simulink model "Mrac_MITS"  (R2015a)
settings: Solver=ode4  StartTime=to  StopTime=tf  FixedStep=dt  RelTol=1e-3
values from neighbouring files (symbols this model uses):
  G = 1/(s+1)    [MRAC_MIT.m]
  gamma1 = 0.5    [MRAC_MIT.m]
  gamma2 = 1    [MRAC_MIT.m]
  gamma3 = 2    [MRAC_MIT.m]
  k = 10* rand(1,length(t))    [MRAC_MIT.m]
libraries: cstblocks x6
settings Model: Creator=dj  LastModifiedBy=dj

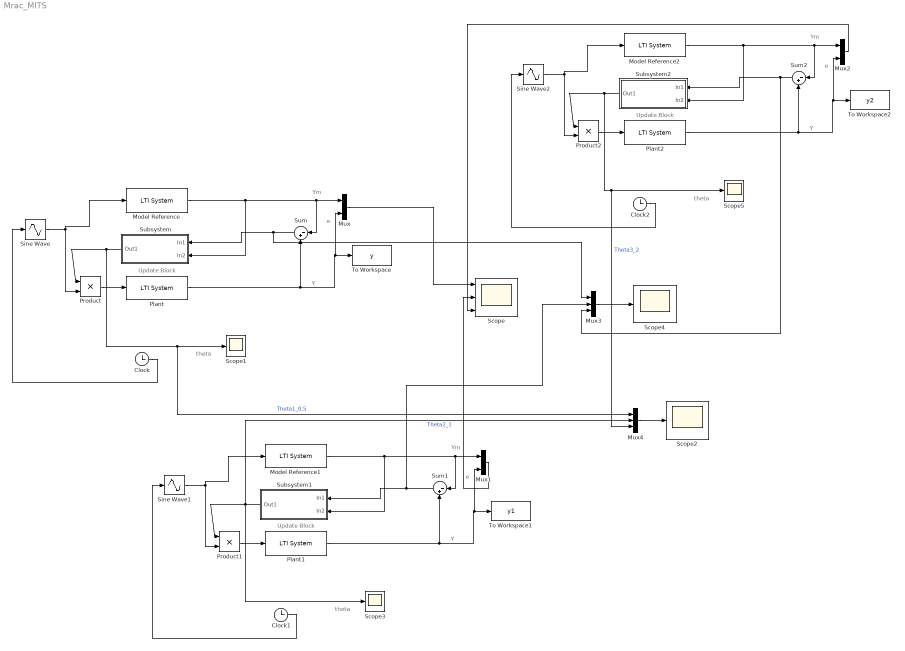
== system Mrac_MITS ==
  note: e
  note: Y
  note: Ym
  note: theta
  note: Update Block
  note: e
  note: Y
  note: Ym
  note: theta
  note: Update Block
  note: e
  note: Y
  note: Ym
  note: theta
  note: Update Block
  Clock : Clock
  Clock1 : Clock
  Clock2 : Clock
  Model Reference : cstblocks/LTI System  sys=Gm  IC=[]
  Model Reference1 : cstblocks/LTI System  sys=Gm  IC=[]
  Model Reference2 : cstblocks/LTI System  sys=Gm  IC=[]
  Mux : Mux  Inputs=2
  Mux1 : Mux  Inputs=2
  Mux2 : Mux  Inputs=2
  Mux3 : Mux  Inputs=3
  Mux4 : Mux  Inputs=3
  Plant : cstblocks/LTI System  sys=k*G  IC=[]
  Plant1 : cstblocks/LTI System  sys=k*G  IC=[]
  Plant2 : cstblocks/LTI System  sys=k*G  IC=[]
  Product : Product
  Product1 : Product
  Product2 : Product
  Scope : Scope  NumInputPorts=3
      settings: YMin=-5~-5~-5  YMax=5~5~5
  Scope{1..5} (5 alike) : Scope
      Scope2 settings: SaveName=ScopeData2
      Scope3 settings: SaveName=ScopeData3
      Scope4 settings: SaveName=ScopeData4
      Scope5 settings: SaveName=ScopeData5
  Sine Wave : Sin  TimeSource=Use external signal  SampleTime=0
  Sine Wave1 : Sin  TimeSource=Use external signal  SampleTime=0
  Sine Wave2 : Sin  TimeSource=Use external signal  SampleTime=0
  Subsystem : Subsystem
  Subsystem1 : Subsystem
  Subsystem2 : Subsystem
  Sum : Sum  Inputs=|-+
  Sum1 : Sum  Inputs=|-+
  Sum2 : Sum  Inputs=|-+
  To Workspace : ToWorkspace  VariableName=y  SaveFormat=Timeseries  SampleTime=-1
  To Workspace1 : ToWorkspace  VariableName=y1  SaveFormat=Timeseries  SampleTime=-1
  To Workspace2 : ToWorkspace  VariableName=y2  SaveFormat=Timeseries  SampleTime=-1
  wires:
  Model Reference/1 -> Subsystem/2(In2), Mux/1, Sum/1
  Product/1 -> Plant/1
  Subsystem/1(Out1) -> Mux4/1, Scope1/1, Product/1  "Theta1_0.5"
  Sum/1 -> Mux3/1, Subsystem/1(In1)
  Sine Wave/1 -> Model Reference/1, Product/2
  Plant/1 -> Mux/2, To Workspace/1, Sum/2
  Clock/1 -> Sine Wave/1
  Model Reference1/1 -> Subsystem1/2(In2), Mux1/1, Sum1/1
  Product1/1 -> Plant1/1
  Subsystem1/1(Out1) -> Mux4/2, Scope3/1, Product1/1  "Theta2_1"
  Sum1/1 -> Mux3/2, Subsystem1/1(In1)
  Sine Wave1/1 -> Model Reference1/1, Product1/2
  Plant1/1 -> Mux1/2, To Workspace1/1, Sum1/2
  Clock1/1 -> Sine Wave1/1
  Model Reference2/1 -> Sum2/1, Mux2/1, Subsystem2/2(In2)
  Product2/1 -> Plant2/1
  Subsystem2/1(Out1) -> Product2/1, Mux4/3, Scope5/1  "Theta3_2"
  Sum2/1 -> Mux3/3, Subsystem2/1(In1)
  Sine Wave2/1 -> Product2/2, Model Reference2/1
  Plant2/1 -> Sum2/2, To Workspace2/1, Mux2/2
  Clock2/1 -> Sine Wave2/1
  Mux2/1 -> Scope/3
  Mux/1 -> Scope/1
  Mux1/1 -> Scope/2
  Mux3/1 -> Scope4/1
  Mux4/1 -> Scope2/1

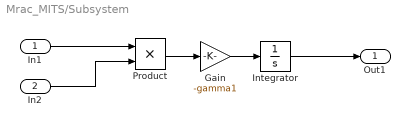
== system Mrac_MITS/Subsystem ==
  In1 : Inport
  In2 : Inport  Port=2
  Gain : Gain  Gain=-gamma1
  Integrator : Integrator
  Product : Product
  Out1 : Outport
  wires:
  In1/1 -> Product/1
  In2/1 -> Product/2
  Product/1 -> Gain/1
  Gain/1 -> Integrator/1
  Integrator/1 -> Out1/1

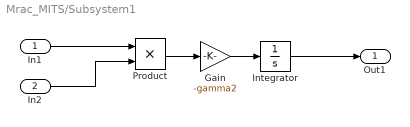
== system Mrac_MITS/Subsystem1 ==
  In1 : Inport
  In2 : Inport  Port=2
  Gain : Gain  Gain=-gamma2
  Integrator : Integrator
  Product : Product
  Out1 : Outport
  wires:
  In1/1 -> Product/1
  In2/1 -> Product/2
  Product/1 -> Gain/1
  Gain/1 -> Integrator/1
  Integrator/1 -> Out1/1

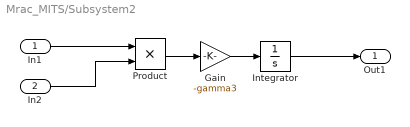
== system Mrac_MITS/Subsystem2 ==
  In1 : Inport
  In2 : Inport  Port=2
  Gain : Gain  Gain=-gamma3
  Integrator : Integrator
  Product : Product
  Out1 : Outport
  wires:
  Integrator/1 -> Out1/1
  Gain/1 -> Integrator/1
  Product/1 -> Gain/1
  In2/1 -> Product/2
  In1/1 -> Product/1
